simulink model "airgap2pos"  (R2022b)
settings: Solver=VariableStepAuto  StartTime=0.0  StopTime=10.0  RelTol=1e-3
settings Model: Creator=USUARIO  LastModifiedBy=USUARIO

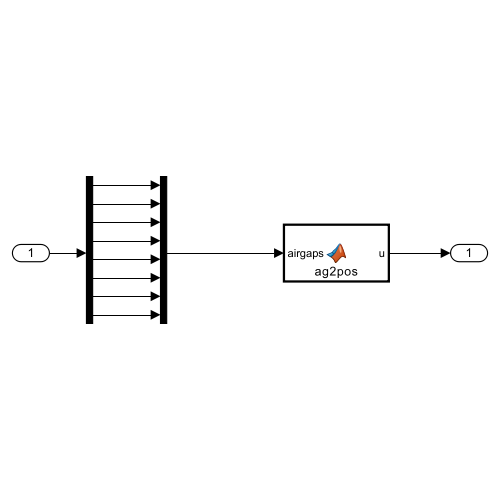
[thumbnail: Simulink's stored preview of the top-level diagram]
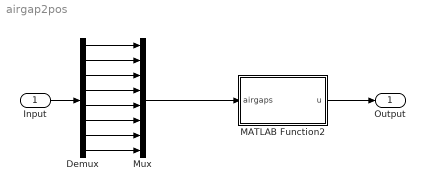
== system airgap2pos ==
  Input : Inport
  Demux : Demux  Outputs=8
  MATLAB Function2 : MATLAB Function  TreatAsAtomicUnit=on
  Mux : Mux  Inputs=8
  Output : Outport
  wires:
  Input/1 -> Demux/1
  MATLAB Function2/1(u) -> Output/1
  Mux/1 -> MATLAB Function2/1(airgaps)
  Demux/1 -> Mux/1
  Demux/2 -> Mux/2
  Demux/3 -> Mux/3
  Demux/4 -> Mux/4
  Demux/5 -> Mux/5
  Demux/6 -> Mux/6
  Demux/7 -> Mux/7
  Demux/8 -> Mux/8

== matlab function airgap2pos/MATLAB Function2 ==
  data: airgaps input; u output
function u = ag2pos(airgaps)

% CONSTANTES

x_sragy = 0.7681; 
y_sragy = 0.0951;
z_sragy = 0.07922; 

x_sragz = 0.76785;
y_sragz = 0.22269;
z_sragz = -0.09493; 

z_infr = 0.6328;

grosorz = 0.015;
grosory = 0.005;

coder.varsize('rotx_aux');
coder.varsize('roty_aux');
coder.varsize('rotz_aux');
coder.varsize('y_aux');
coder.varsize('z_aux');

rotx_aux=zeros(2,1);
roty_aux=zeros(2,1);
rotz_aux=zeros(2,1);
y_aux=zeros(4,1);
z_aux=zeros(4,1);

% ROTACIONES
rotx_aux(1) = asin((airgaps(2) - airgaps(1))/(2*y_sragz));
rotx_aux(2) = asin((airgaps(4) - airgaps(3))/(2*y_sragz));

roty_aux(1) = asin((airgaps(1) - airgaps(3))/(2*x_sragz));
roty_aux(2) = asin((airgaps(2) - airgaps(4))/(2*x_sragz));

rotz_aux(1) = asin((airgaps(5) - airgaps(7))/(2*x_sragy));
rotz_aux(2) = asin((airgaps(8) - airgaps(6))/(2*x_sragy));

rotx = mean(rotx_aux);
roty = mean(roty_aux);
rotz = mean(rotz_aux);

% DISTANCIAS
y_aux(1) = + airgaps(5) - y_sragy * cos(rotz) - x_sragy * sin(rotz) + y_sragz * sin(rotx);
y_aux(2) = - airgaps(6) + y_sragy * cos(rotz) - x_sragy * sin(rotz) + y_sragz * sin(rotx);
y_aux(3) = + airgaps(7) - y_sragy * cos(rotz) + x_sragy * sin(rotz) + y_sragz * sin(rotx);
y_aux(4) = - airgaps(8) + y_sragy * cos(rotz) + x_sragy * sin(rotz) + y_sragz * sin(rotx);

z_aux(1) = z_infr - airgaps(1) - z_sragz * cos(roty) + x_sragz * sin(roty) - y_sragz * sin(rotx);
z_aux(2) = z_infr - airgaps(2) - z_sragz * cos(roty) + x_sragz * sin(roty) + y_sragz * sin(rotx);
z_aux(3) = z_infr - airgaps(3) - z_sragz * cos(roty) - x_sragz * sin(roty) - y_sragz * sin(rotx);
z_aux(4) = z_infr - airgaps(4) - z_sragz * cos(roty) - x_sragz * sin(roty) + y_sragz * sin(rotx);



y = mean(y_aux);
z = mean(z_aux);

u =[y, z, rotx, roty, rotz]';
